simulink model "simpleSuperStep"  (R2023a)
settings: Solver=FixedStepDiscrete  StartTime=0.0  StopTime=10.0  RelTol=1e-3  EnableMultiTasking=on
undefined symbols (not defined in the file): sigbuilder_block
settings Model: Creator=jrivitus  LastModifiedBy=Administrator
settings SolverCC: ZeroCrossAlgorithm=Non-adaptive  AlgebraicLoopSolver=TrustRegion
settings DataIOCC: LimitDataPoints=on  SaveFormat=Array  SignalLoggingSaveFormat=ModelDataLogs  ReturnWorkspaceOutputs=off
settings OptimizationCC: ExpressionDepthLimit=2147483647  InitFltsAndDblsToZero=on  LifeSpan=inf
settings DebuggingCC: UnderspecifiedInitializationDetection=Classic  MergeDetectMultiDrivingBlocksExec=none  FcnCallInpInsideContextMsg=warning  UnconnectedInputMsg=warning  UnconnectedOutputMsg=warning  UnconnectedLineMsg=warning  StateNameClashWarn=warning  SFUnexpectedBacktrackingDiag=warning  SFNoUnconditionalDefaultTransitionDiag=warning  SFExecutionAtInitializationDiag=none  ArithmeticOperatorsInVariantConditions=warning
settings HardwareCC: ProdBitPerPointer=32  ProdBitPerSizeT=32  ProdBitPerPtrDiffT=32  ProdLargestAtomicFloat=None  ProdIntDivRoundTo=Undefined  ProdEndianess=Unspecified  ProdWordSize=32  ProdHWDeviceType=32-bit Generic
settings ModelReferenceCC: PropagateSignalLabelsOutOfModel=off
settings SFSimCC: SimParseCustomCode=off
settings CodeAppCC: StateflowObjectComments=on
settings GRTTargetCC: TargetLangStandard=C89/C90 (ANSI)  CombineOutputUpdateFcns=off  GRTInterface=on
settings ConfigComp: CovMetricSettings=dw  CovSaveCumulativeToWorkspaceVar=on  CovSaveSingleToWorkspaceVar=on

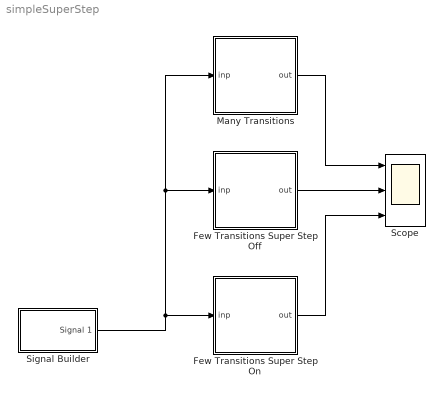
== system simpleSuperStep ==
  Few Transitions Super Step Off : Stateflow chart  TreatAsAtomicUnit=on
  Few Transitions Super Step On : Stateflow chart  TreatAsAtomicUnit=on
  Many Transitions : Stateflow chart  TreatAsAtomicUnit=on
  Scope : Scope  NumInputPorts=3
  Signal Builder : Subsystem  Tag=STV Subsys  LoadFcn=sigbuilder_block('load');  StartFcn=sigbuilder_block('start');  StopFcn=sigbuilder_block('stop');  ClipboardFcn=sigbuilder_block('clipboard');  mask(Sigbuilder block){tuvar=[0:10]}
      mask help: Sigbuilder GUI
      mask init:
      | if ~strcmp(get_param(bdroot(gcbh),'SimulationStatus'),'stopped') tuvar = sigbuilder_block('maskInit'); end
      settings: CopyFcn=sigbuilder_block('copy');  DeleteFcn=sigbuilder_block('delete');  ModelCloseFcn=sigbuilder_block('modelClose');  PreSaveFcn=sigbuilder_block('preSave');  PauseFcn=sigbuilder_block('pause')  ContinueFcn=sigbuilder_block('continue')  NameChangeFcn=sigbuilder_block('namechange');  OpenFcn=sigbuilder_block('open',[309.6 71.4 550.2 400.2 ]);  CloseFcn=sigbuilder_block('close');
      mask Display: plot(0, 0, 100, 100,[2, 2, 32, 32, 2], [68, 8, 8, 68, 68],[32, 2], [38, 38], [32, 19, 2],[53, 60, 44], [32, 17, 17, 2],[16, 16, 31, 31]);txt = getActiveGroup(gcbh);text(2, 100, txt,'verticalAlignment', 'top');
  wires:
  Signal Builder/1(Signal 1) -> Many Transitions/1(inp), Few Transitions Super Step Off/1(inp), Few Transitions Super Step On/1(inp)
  Many Transitions/1(out) -> Scope/1
  Few Transitions Super Step Off/1(out) -> Scope/2
  Few Transitions Super Step On/1(out) -> Scope/3

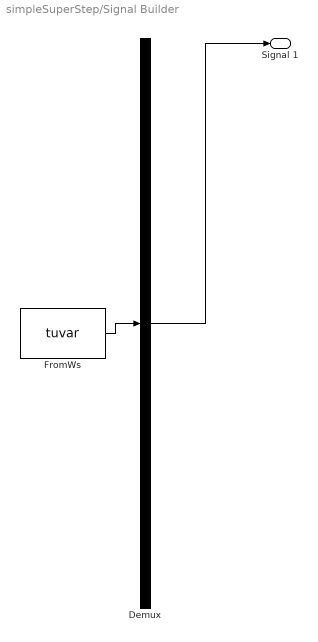
== system simpleSuperStep/Signal Builder ==
  Demux : Demux  Tag=STV Demux  Outputs=1
      settings: DisplayOption=none
  FromWs : FromWorkspace  Tag=STV FromWs  VariableName=tuvar
      SigBuilderData=|
      | common.afterFinalStr = 'Extrapolate'
      | common.sampleTime = 0
      | dataSet.timeRange = [0 10]
      | dataSet.name = 'Group 1'
      | sbobj.Name = 'Signal Builder'
      | sbobj.Groups.Name = 'Group 1'
      | sbobj.Groups.Signals.Name = 'Signal 1'
      | sbobj.Groups.Signals.XData = [0 2 2 4 4 6 6 8 8 10]
      | sbobj.Groups.Signals.YData = [0 0 6.05 6.05 0 0 11 11 0 0]
  Signal 1 : Outport  Tag=STV Outport
  wires:
  Demux/1 -> Signal 1/1
  FromWs/1 -> Demux/1

== stateflow chart simpleSuperStep/Many Transitions ==
  state A
    en: out = 0;
  state B
    en: out = 2;
  state C
    en: out = 5;
  A -> C [order 1] : [inp > 10]
  (default) -> A
  B -> C [order 1] : [inp > 10]
  A -> B [order 2] : [inp > 5]
  C -> B [order 2] : [inp <= 10]
  B -> A [order 2] : [inp <= 5]
  C -> A [order 1] : [inp <= 5]
  data: inp input; out output double

== stateflow chart simpleSuperStep/Few Transitions Super Step Off ==
  state A
    en: out = 0;
  state B
    en: out = 2;
  state C
    en: out = 5;
  (default) -> A
  B -> C [order 1] : [inp > 10]
  A -> B : [inp > 5]
  C -> B : [inp <= 10]
  B -> A [order 2] : [inp <= 5]
  data: inp input; out output double

== stateflow chart simpleSuperStep/Few Transitions Super Step On ==
  settings: enableNonTerminalStates=1
  state A
    en: out = 1;
  state B
    en: out = 2;
  state C
    en: out = 3;
  (default) -> A
  B -> C [order 1] : [inp > 10]
  A -> B : [inp > 5]
  C -> B : [inp <= 10]
  B -> A [order 2] : [inp <= 5]
  data: inp input; out output double
